simulink model "ExistingSISOmodeling"  (R2020a)
settings: Solver=VariableStepAuto  StartTime=0.0  StopTime=15000  RelTol=1e-3
undefined symbols (not defined in the file): Kd
libraries: cstblocks x2
settings Model: Creator=User  LastModifiedBy=User
settings SolverCC: AlgebraicLoopSolver=LineSearch

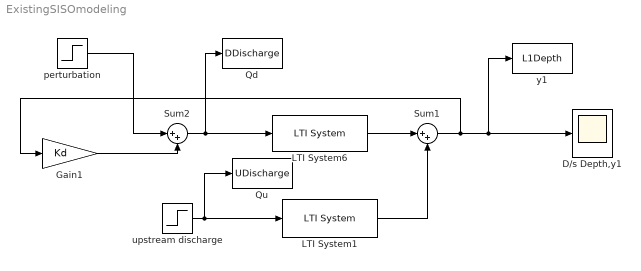
== system ExistingSISOmodeling ==
  D/s Depth,y1 : Scope
  Gain1 : Gain  Gain=Kd
  LTI System1 : cstblocks/LTI System  sys=P21  IC=[]
  LTI System6 : cstblocks/LTI System  sys=P22  IC=[]
  Qd : ToWorkspace  VariableName=DDischarge  SaveFormat=Timeseries  SampleTime=-1
  Qu : ToWorkspace  VariableName=UDischarge  SaveFormat=Timeseries  SampleTime=-1
  Sum1 : Sum  Inputs=|++
  Sum2 : Sum  Inputs=|++
  perturbation : Step  Time=1200  After=0.15  SampleTime=0
  upstream discharge : Step  Time=1200  After=0  SampleTime=0
  y1 : ToWorkspace  VariableName=L1Depth  SaveFormat=Timeseries  SampleTime=-1
  wires:
  LTI System6/1 -> Sum1/1
  Gain1/1 -> Sum2/2
  Sum1/1 -> Gain1/1, D/s Depth,y1/1, y1/1
  Sum2/1 -> LTI System6/1, Qd/1
  perturbation/1 -> Sum2/1
  LTI System1/1 -> Sum1/2
  upstream discharge/1 -> LTI System1/1, Qu/1
